simulink model "Environment_Model"  (R2016b)
settings: Solver=FixedStepDiscrete  StartTime=0.0  StopTime=inf  FixedStep=EnvMdl.tiSimnTiStep_C.Value  RelTol=1e-3  EnableMultiTasking=on
InitFcn:
  | % Call parameters initialization function
  | % run optiTruck_init_sim.m;
StopFcn:
  | %optiTruck_post_sim;
  | %optiTruck_plot_sim;
undefined symbols (not defined in the file or in its folder): gui_data
settings Model: Creator=engin  LastModifiedBy=engin.ozatay
settings DataIOCC: SaveFormat=StructureWithTime  SaveOutput=off  DSMLogging=off  VisualizeSimOutput=off  SaveTime=off  SignalLoggingName=Results
settings OptimizationCC: BlockReduction=off  ConditionallyExecuteInputs=off  LifeSpan=inf
settings DebuggingCC: AllowSymbolicDim=off  SFUnexpectedBacktrackingDiag=warning  SFNoUnconditionalDefaultTransitionDiag=warning  SFExecutionAtInitializationDiag=none
settings ModelReferenceCC: ModelReferenceNumInstancesAllowed=Single  PropagateSignalLabelsOutOfModel=off
settings GRTTargetCC: TargetLangStandard=C89/C90 (ANSI)
settings ConfigComp: CovMetricSettings=dw  CovHtmlReporting=on  CovSaveCumulativeToWorkspaceVar=on  CovSaveSingleToWorkspaceVar=on  CovExternalEMLEnable=off

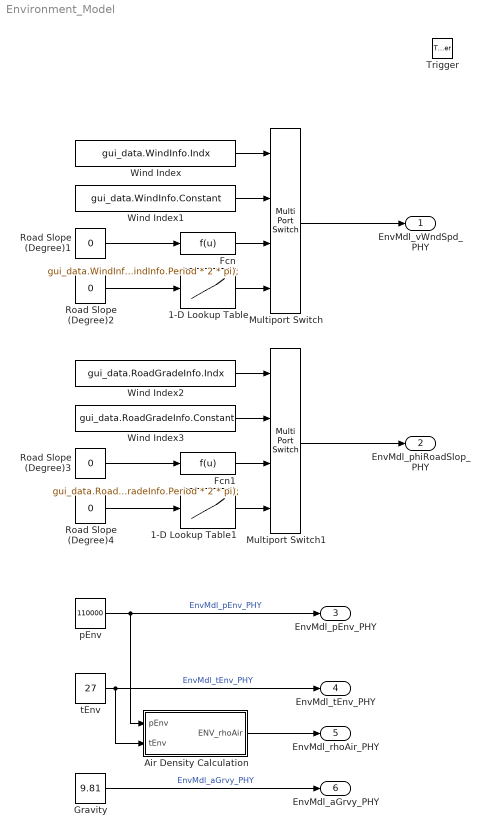
== system Environment_Model ==
  Trigger : TriggerPort  TriggerType=function-call  VariantControl=Variant  PortDimensions=1
  1-D Lookup Table : Lookup_n-D  NumberOfTableDimensions=1  BreakpointsForDimension1=gui_data.RouteInfo.Distance  Table=gui_data.RouteInfo.Wind  InternalRulePriority=Speed  RndMeth=Simplest  InputSameDT=on
  1-D Lookup Table1 : Lookup_n-D  NumberOfTableDimensions=1  BreakpointsForDimension1=gui_data.RouteInfo.Distance  Table=gui_data.RouteInfo.Grade  InternalRulePriority=Speed  RndMeth=Simplest  InputSameDT=on
  Air Density Calculation : Subsystem
  Fcn : Fcn  Expr=gui_data.WindInfo.Amplitude*sin(u(1)/gui_data.WindInfo.Period * 2 * pi);
  Fcn1 : Fcn  Expr=gui_data.RoadGradeInfo.Amplitude*sin(u(1)/gui_data.RoadGradeInfo.Period * 2 * pi);
  Gravity : Constant  Value=9.81  SampleTime=-1
  Multiport Switch : MultiPortSwitch
  Multiport Switch1 : MultiPortSwitch
  Road Slope (Degree){1..4} (4 alike) : Constant  Value=0  SampleTime=-1
  Wind Index : Constant  Value=gui_data.WindInfo.Indx  SampleTime=-1
  Wind Index1 : Constant  Value=gui_data.WindInfo.Constant  SampleTime=-1
  Wind Index2 : Constant  Value=gui_data.RoadGradeInfo.Indx  SampleTime=-1
  Wind Index3 : Constant  Value=gui_data.RoadGradeInfo.Constant  SampleTime=-1
  pEnv : Constant  Value=110000  SampleTime=-1
  tEnv : Constant  Value=27  SampleTime=-1
  EnvMdl_vWndSpd_PHY : Outport
  EnvMdl_phiRoadSlop_PHY : Outport  Port=2
  EnvMdl_pEnv_PHY : Outport  Port=3
  EnvMdl_tEnv_PHY : Outport  Port=4
  EnvMdl_rhoAir_PHY : Outport  Port=5
  EnvMdl_aGrvy_PHY : Outport  Port=6
  wires:
  pEnv/1 -> Air Density Calculation/1(pEnv), EnvMdl_pEnv_PHY/1  "EnvMdl_pEnv_PHY"
  tEnv/1 -> Air Density Calculation/2(tEnv), EnvMdl_tEnv_PHY/1  "EnvMdl_tEnv_PHY"
  Gravity/1 -> EnvMdl_aGrvy_PHY/1  "EnvMdl_aGrvy_PHY"
  Air Density Calculation/1(ENV_rhoAir) -> EnvMdl_rhoAir_PHY/1
  Wind Index/1 -> Multiport Switch/1
  Wind Index1/1 -> Multiport Switch/2
  Fcn/1 -> Multiport Switch/3
  Road Slope (Degree)1/1 -> Fcn/1
  1-D Lookup Table/1 -> Multiport Switch/4
  Road Slope (Degree)2/1 -> 1-D Lookup Table/1
  Road Slope (Degree)3/1 -> Fcn1/1
  Road Slope (Degree)4/1 -> 1-D Lookup Table1/1
  Wind Index2/1 -> Multiport Switch1/1
  Wind Index3/1 -> Multiport Switch1/2
  Fcn1/1 -> Multiport Switch1/3
  1-D Lookup Table1/1 -> Multiport Switch1/4
  Multiport Switch/1 -> EnvMdl_vWndSpd_PHY/1
  Multiport Switch1/1 -> EnvMdl_phiRoadSlop_PHY/1

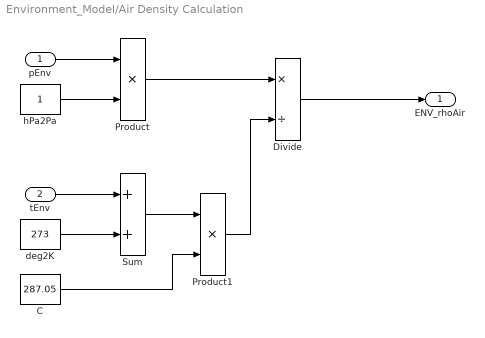
== system Environment_Model/Air Density Calculation ==
  pEnv : Inport
  tEnv : Inport  Port=2
  C : Constant  Value=287.05  SampleTime=-1
  Divide : Product  Inputs=*/
  Product : Product  RndMeth=Zero
  Product1 : Product  RndMeth=Zero
  Sum : Sum
  deg2K : Constant  Value=273  SampleTime=-1
  hPa2Pa : Constant  SampleTime=-1
  ENV_rhoAir : Outport
  wires:
  Divide/1 -> ENV_rhoAir/1
  Product1/1 -> Divide/2
  C/1 -> Product1/2
  Sum/1 -> Product1/1
  deg2K/1 -> Sum/2
  tEnv/1 -> Sum/1
  Product/1 -> Divide/1
  hPa2Pa/1 -> Product/2
  pEnv/1 -> Product/1
